simulink library "SignalGeneratorLibBtc"  (R2022b)
settings: Solver=VariableStepAuto  StartTime=0.0  StopTime=10.0  RelTol=1e-3
libraries: simulink x16, FeaturePath x6, HandyTextFile x6, RTC x6, TuneVar x1
(part 2 of 2)

== system SignalGeneratorLibBtc/WhiteNoiseGen/ForEachSubsystem/SimulationTimeTriggered_Subsystem ==
  Constant : Constant  SampleTime=-1
  Digital Clock : DigitalClock  SampleTime=-1
  Equal : RelationalOperator  Operator===  OutDataTypeStr=boolean  RndMeth=Simplest  InputSameDT=off
  SimuliationTimeTriggerdOut1 : Outport  VectorParamsAs1DForOutWhenUnconnected=off
  wires:
  Equal/1 -> SimuliationTimeTriggerdOut1/1
  Constant/1 -> Equal/1
  Digital Clock/1 -> Equal/2

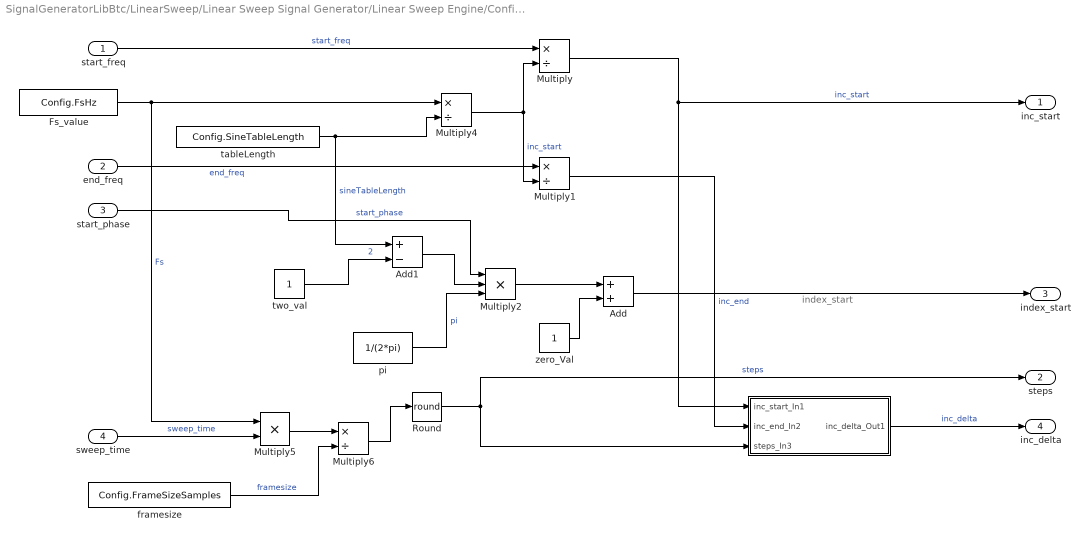
== system SignalGeneratorLibBtc/LinearSweep/Linear Sweep Signal Generator/Linear Sweep Engine/Configuration_sublock ==
  note: index_start
  start_freq : Inport
  end_freq : Inport  Port=2
  start_phase : Inport  Port=3
  "sweep_time " : Inport  Port=4
  " " : Subsystem  TreatAsAtomicUnit=on
  Add : Sum
  Add1 : Sum  Inputs=+-
  Fs_value : Constant  Value=Config.FsHz  OutDataTypeStr=single
  Multiply{,1,4,6} (4 alike) : Product  Inputs=*/
  Multiply2 : Product  Inputs=***
  Multiply5 : Product  Inputs=**
  Round : Rounding  Operator=round
  framesize : Constant  Value=Config.FrameSizeSamples  VectorParams1D=off  OutDataTypeStr=uint32
  pi : Constant  Value=1/(2*pi)  VectorParams1D=off  OutDataTypeStr=single
  tableLength : Constant  Value=Config.SineTableLength  VectorParams1D=off  OutDataTypeStr=single
  two_val : Constant  VectorParams1D=off  OutDataTypeStr=uint32
  zero_Val : Constant  VectorParams1D=off  OutDataTypeStr=single
  inc_start : Outport  VectorParamsAs1DForOutWhenUnconnected=off
  steps : Outport  Port=2  VectorParamsAs1DForOutWhenUnconnected=off
  index_start : Outport  Port=3  VectorParamsAs1DForOutWhenUnconnected=off
  inc_delta : Outport  Port=4  VectorParamsAs1DForOutWhenUnconnected=off
  wires:
  " "/1(inc_delta_Out1) -> inc_delta/1  "inc_delta"
  Round/1 -> steps/1, " "/3(steps_In3)  "steps"
  Multiply6/1 -> Round/1
  framesize/1 -> Multiply6/2  "framesize"
  Multiply5/1 -> Multiply6/1
  "sweep_time "/1 -> Multiply5/2  "sweep_time"
  Multiply1/1 -> " "/2(inc_end_In2)  "inc_end"
  Multiply4/1 -> Multiply/2, Multiply1/2  "inc_start"
  Multiply/1 -> inc_start/1, " "/1(inc_start_In1)  "inc_start"
  Add/1 -> index_start/1
  end_freq/1 -> Multiply1/1  "end_freq"
  start_phase/1 -> Multiply2/1  "start_phase"
  start_freq/1 -> Multiply/1  "start_freq"
  tableLength/1 -> Add1/1, Multiply4/2  "sineTableLength"
  Multiply2/1 -> Add/1
  Fs_value/1 -> Multiply4/1, Multiply5/1  "Fs"
  pi/1 -> Multiply2/3  "pi"
  two_val/1 -> Add1/2  "2"
  zero_Val/1 -> Add/2
  Add1/1 -> Multiply2/2

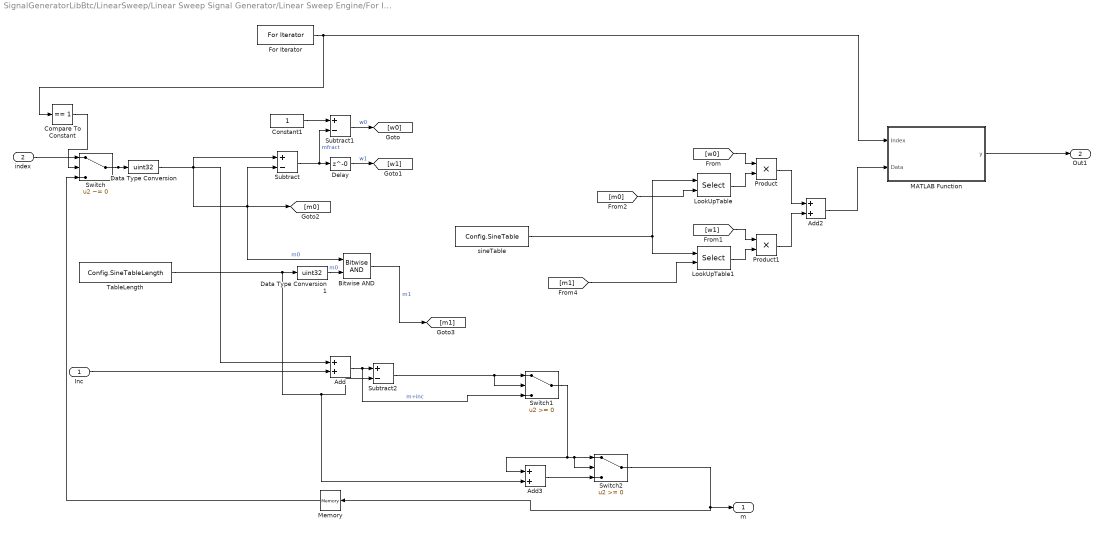
== system SignalGeneratorLibBtc/LinearSweep/Linear Sweep Signal Generator/Linear Sweep Engine/For Iterator Subsystem ==
  "Inc " : Inport
  index : Inport  Port=2
  Add : Sum
  Add2 : Sum
  Add3 : Sum
  Bitwise AND : simulink/Logic and Bit Operations/Bitwise Operator  logicop=AND  UseBitMask=off  NumInputPorts=2  BitMask=bin2dec('11011001')  BitMaskRealWorld=Stored Integer
  Compare To Constant : simulink/Logic and Bit Operations/Compare To Constant  relop===  const=1  OutDataTypeStr=boolean
  Constant1 : Constant  OutDataTypeStr=single
  Data Type Conversion : DataTypeConversion  OutDataTypeStr=uint32  SaturateOnIntegerOverflow=off  RndMeth=Floor
  Data Type Conversion1 : DataTypeConversion  OutDataTypeStr=uint32  SaturateOnIntegerOverflow=off  RndMeth=Floor
  Delay : Delay  DelayLength=0
  For Iterator : ForIterator  ResetStates=reset  IterationLimit=Config.FrameSizeSamples
  LookUpTable : Selector  IndexMode=Zero-based  InputPortWidth=Config.SineTableLength  IndexOptions=Index vector (port)  Indices=[1 3]  OutputSizes=1
  LookUpTable1 : Selector  IndexMode=Zero-based  InputPortWidth=Config.SineTableLength  IndexOptions=Index vector (port)  Indices=[1 3]  OutputSizes=1
  MATLAB Function : MATLAB Function  TreatAsAtomicUnit=on  mask{Nch=Config.NumChannel, frameSize_samples=Config.FrameSizeSamples}
  Memory : Memory  InheritSampleTime=on
  Product : Product
  Product1 : Product
  Subtract : Sum  Inputs=+-  OutDataTypeStr=single
  Subtract1 : Sum  Inputs=+-  OutDataTypeStr=single
  Subtract2 : Sum  Inputs=+-
  Switch : Switch  Criteria=u2 ~= 0  SaturateOnIntegerOverflow=off  InputSameDT=off
  Switch1 : Switch  SaturateOnIntegerOverflow=off  InputSameDT=off
  Switch2 : Switch  SaturateOnIntegerOverflow=off  InputSameDT=off
  TableLength : Constant  Value=Config.SineTableLength  VectorParams1D=off  OutDataTypeStr=single
  sineTable : Constant  Value=Config.SineTable  VectorParams1D=off  OutDataTypeStr=single
  m : Outport  VectorParamsAs1DForOutWhenUnconnected=off
  Out1 : Outport  Port=2  VectorParamsAs1DForOutWhenUnconnected=off
  wires:
  TableLength/1 -> Data Type Conversion1/1, Add3/2, Subtract2/2
  Compare To Constant/1 -> Switch/2
  index/1 -> Switch/1
  Switch/1 -> Add/1, Data Type Conversion/1
  Add/1 -> Switch1/3, Subtract2/1  "m+inc"
  For Iterator/1 -> Compare To Constant/1, MATLAB Function/1(Index)
  Memory/1 -> Switch/3
  Data Type Conversion/1 -> Bitwise AND/1, Subtract/2, [m0], Subtract/1  "m0"
  Subtract/1 -> Delay/1, Subtract1/2  "mfract"
  Constant1/1 -> Subtract1/1
  Subtract1/1 -> [w0]  "w0"
  Delay/1 -> [w1]  "w1"
  sineTable/1 -> LookUpTable1/1, LookUpTable/1
  [m0] -> LookUpTable/2
  [w0] -> Product/1
  LookUpTable/1 -> Product/2
  [m1] -> LookUpTable1/2
  [w1] -> Product1/1
  LookUpTable1/1 -> Product1/2
  Product/1 -> Add2/1
  Product1/1 -> Add2/2
  MATLAB Function/1(y) -> Out1/1
  "Inc "/1 -> Add/2
  Data Type Conversion1/1 -> Bitwise AND/2  "m0"
  Switch1/1 -> Add3/1, Switch2/2, Switch2/1
  Switch2/1 -> Memory/1, m/1
  Subtract2/1 -> Switch1/1, Switch1/2
  Add3/1 -> Switch2/3
  Bitwise AND/1 -> [m1]  "m1"
  Add2/1 -> MATLAB Function/2(Data)

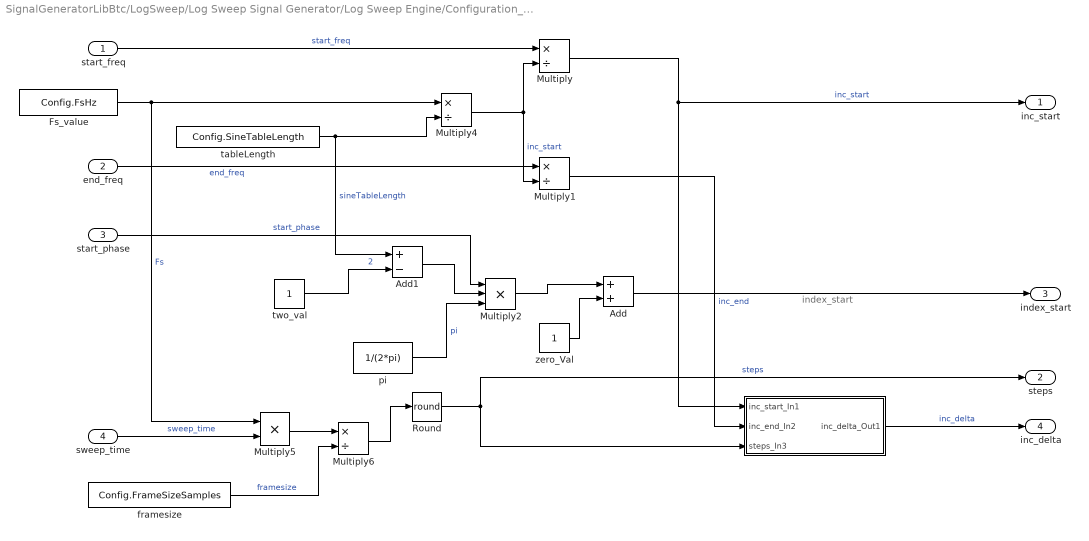
== system SignalGeneratorLibBtc/LogSweep/Log Sweep Signal Generator/Log Sweep Engine/Configuration_sublock ==
  note: index_start
  start_freq : Inport
  end_freq : Inport  Port=2
  start_phase : Inport  Port=3
  "sweep_time " : Inport  Port=4
  " " : Subsystem  AncestorBlock=SignalGenerator/LogSweep/Log Sweep Signal Generator/Log Sweep Engine/Log_Sweep_Subsystem/Configuration_sublock/  TreatAsAtomicUnit=on
      settings: LibrarySourceBlock=SignalGenerator/LogSweep/Log Sweep Signal Generator/Log Sweep Engine/Log_Sweep_Subsystem/Configuration_sublock/
  Add : Sum
  Add1 : Sum  Inputs=+-
  Fs_value : Constant  Value=Config.FsHz  OutDataTypeStr=single
  Multiply{,1,4,6} (4 alike) : Product  Inputs=*/
  Multiply2 : Product  Inputs=***
  Multiply5 : Product  Inputs=**
  Round : Rounding  Operator=round
  framesize : Constant  Value=Config.FrameSizeSamples  VectorParams1D=off  OutDataTypeStr=uint32
  pi : Constant  Value=1/(2*pi)  VectorParams1D=off  OutDataTypeStr=single
  tableLength : Constant  Value=Config.SineTableLength  VectorParams1D=off  OutDataTypeStr=single
  two_val : Constant  VectorParams1D=off  OutDataTypeStr=uint32
  zero_Val : Constant  VectorParams1D=off  OutDataTypeStr=single
  inc_start : Outport  VectorParamsAs1DForOutWhenUnconnected=off
  steps : Outport  Port=2  VectorParamsAs1DForOutWhenUnconnected=off
  index_start : Outport  Port=3  VectorParamsAs1DForOutWhenUnconnected=off
  inc_delta : Outport  Port=4  VectorParamsAs1DForOutWhenUnconnected=off
  wires:
  " "/1(inc_delta_Out1) -> inc_delta/1  "inc_delta"
  Round/1 -> steps/1, " "/3(steps_In3)  "steps"
  Multiply6/1 -> Round/1
  framesize/1 -> Multiply6/2  "framesize"
  Multiply5/1 -> Multiply6/1
  "sweep_time "/1 -> Multiply5/2  "sweep_time"
  Multiply1/1 -> " "/2(inc_end_In2)  "inc_end"
  Multiply4/1 -> Multiply/2, Multiply1/2  "inc_start"
  Multiply/1 -> inc_start/1, " "/1(inc_start_In1)  "inc_start"
  Add/1 -> index_start/1
  end_freq/1 -> Multiply1/1  "end_freq"
  start_freq/1 -> Multiply/1  "start_freq"
  Multiply2/1 -> Add/1
  Fs_value/1 -> Multiply4/1, Multiply5/1  "Fs"
  zero_Val/1 -> Add/2
  Add1/1 -> Multiply2/2
  pi/1 -> Multiply2/3  "pi"
  two_val/1 -> Add1/2  "2"
  tableLength/1 -> Add1/1, Multiply4/2  "sineTableLength"
  start_phase/1 -> Multiply2/1  "start_phase"

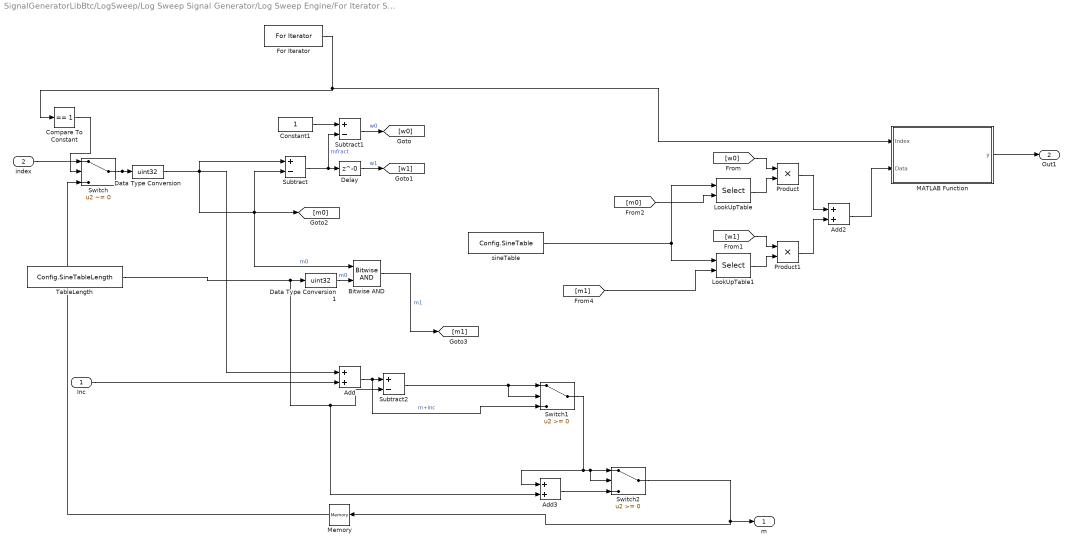
== system SignalGeneratorLibBtc/LogSweep/Log Sweep Signal Generator/Log Sweep Engine/For Iterator Subsystem ==
  "Inc " : Inport
  index : Inport  Port=2
  Add : Sum
  Add2 : Sum
  Add3 : Sum
  Bitwise AND : simulink/Logic and Bit Operations/Bitwise Operator  logicop=AND  UseBitMask=off  NumInputPorts=2  BitMask=bin2dec('11011001')  BitMaskRealWorld=Stored Integer
  Compare To Constant : simulink/Logic and Bit Operations/Compare To Constant  relop===  const=1  OutDataTypeStr=boolean
  Constant1 : Constant  OutDataTypeStr=single
  Data Type Conversion : DataTypeConversion  OutDataTypeStr=uint32  SaturateOnIntegerOverflow=off  RndMeth=Floor
  Data Type Conversion1 : DataTypeConversion  OutDataTypeStr=uint32  SaturateOnIntegerOverflow=off  RndMeth=Floor
  Delay : Delay  DelayLength=0
  For Iterator : ForIterator  ResetStates=reset  IterationLimit=Config.FrameSizeSamples
  LookUpTable : Selector  IndexMode=Zero-based  InputPortWidth=Config.SineTableLength  IndexOptions=Index vector (port)  Indices=[1 3]  OutputSizes=1
  LookUpTable1 : Selector  IndexMode=Zero-based  InputPortWidth=Config.SineTableLength  IndexOptions=Index vector (port)  Indices=[1 3]  OutputSizes=1
  MATLAB Function : MATLAB Function  TreatAsAtomicUnit=on  mask{Nch=Config.NumChannel, frameSize_samples=Config.FrameSizeSamples}
  Memory : Memory  InheritSampleTime=on
  Product : Product
  Product1 : Product
  Subtract : Sum  Inputs=+-  OutDataTypeStr=single
  Subtract1 : Sum  Inputs=+-  OutDataTypeStr=single
  Subtract2 : Sum  Inputs=+-
  Switch : Switch  Criteria=u2 ~= 0  SaturateOnIntegerOverflow=off  InputSameDT=off
  Switch1 : Switch  SaturateOnIntegerOverflow=off  InputSameDT=off
  Switch2 : Switch  SaturateOnIntegerOverflow=off  InputSameDT=off
  TableLength : Constant  Value=Config.SineTableLength  VectorParams1D=off  OutDataTypeStr=single
  sineTable : Constant  Value=Config.SineTable  VectorParams1D=off  OutDataTypeStr=single
  m : Outport  VectorParamsAs1DForOutWhenUnconnected=off
  Out1 : Outport  Port=2  VectorParamsAs1DForOutWhenUnconnected=off
  wires:
  TableLength/1 -> Data Type Conversion1/1, Add3/2, Subtract2/2
  Compare To Constant/1 -> Switch/2
  index/1 -> Switch/1
  Switch/1 -> Add/1, Data Type Conversion/1
  Add/1 -> Switch1/3, Subtract2/1  "m+inc"
  For Iterator/1 -> MATLAB Function/1(Index), Compare To Constant/1
  Memory/1 -> Switch/3
  Data Type Conversion/1 -> Bitwise AND/1, Subtract/2, [m0], Subtract/1  "m0"
  Subtract/1 -> Delay/1, Subtract1/2  "mfract"
  Constant1/1 -> Subtract1/1
  Subtract1/1 -> [w0]  "w0"
  Delay/1 -> [w1]  "w1"
  sineTable/1 -> LookUpTable1/1, LookUpTable/1
  [m0] -> LookUpTable/2
  [w0] -> Product/1
  LookUpTable/1 -> Product/2
  [m1] -> LookUpTable1/2
  [w1] -> Product1/1
  LookUpTable1/1 -> Product1/2
  Product/1 -> Add2/1
  Product1/1 -> Add2/2
  MATLAB Function/1(y) -> Out1/1
  "Inc "/1 -> Add/2
  Data Type Conversion1/1 -> Bitwise AND/2  "m0"
  Switch1/1 -> Add3/1, Switch2/2, Switch2/1
  Switch2/1 -> Memory/1, m/1
  Subtract2/1 -> Switch1/1, Switch1/2
  Add3/1 -> Switch2/3
  Bitwise AND/1 -> [m1]  "m1"
  Add2/1 -> MATLAB Function/2(Data)

== system SignalGeneratorLibBtc/MultiToneGen/Multitone Signal Generator/Multitone Engine/Configuration_sublock ==
  note: index_start
  start_freq : Inport
  start_phase : Inport  Port=2
  Add : Sum
  Fs_value : Constant  Value=Config.FsHz  OutDataTypeStr=single
  Incdelta : Constant  Value=0  OutDataTypeStr=uint32
  Multiply : Product  Inputs=*/
  Multiply1 : Product  Inputs=***
  Multiply4 : Product  Inputs=*/
  Subtract : Sum  Inputs=+-
  constant2 : Constant  OutDataTypeStr=uint32
  tableLength : Constant  Value=Config.SineTableLength  OutDataTypeStr=single
  two_val : Constant  Value=1/(2*pi)  OutDataTypeStr=single
  inc_start : Outport  VectorParamsAs1DForOutWhenUnconnected=off
  index_start : Outport  Port=2  VectorParamsAs1DForOutWhenUnconnected=off
  inc_delta : Outport  Port=3  VectorParamsAs1DForOutWhenUnconnected=off
  wires:
  Incdelta/1 -> inc_delta/1  "inc_delta"
  Multiply4/1 -> Multiply/2
  Multiply/1 -> inc_start/1  "inc_start"
  Add/1 -> index_start/1
  start_phase/1 -> Multiply1/1  "start_phase"
  start_freq/1 -> Multiply/1  "start_freq"
  Multiply1/1 -> Add/1
  tableLength/1 -> Subtract/1, Multiply4/2  "sineTableLength"
  Fs_value/1 -> Multiply4/1  "Fs"
  two_val/1 -> Multiply1/3  "2"
  constant2/1 -> Add/2, Subtract/2
  Subtract/1 -> Multiply1/2

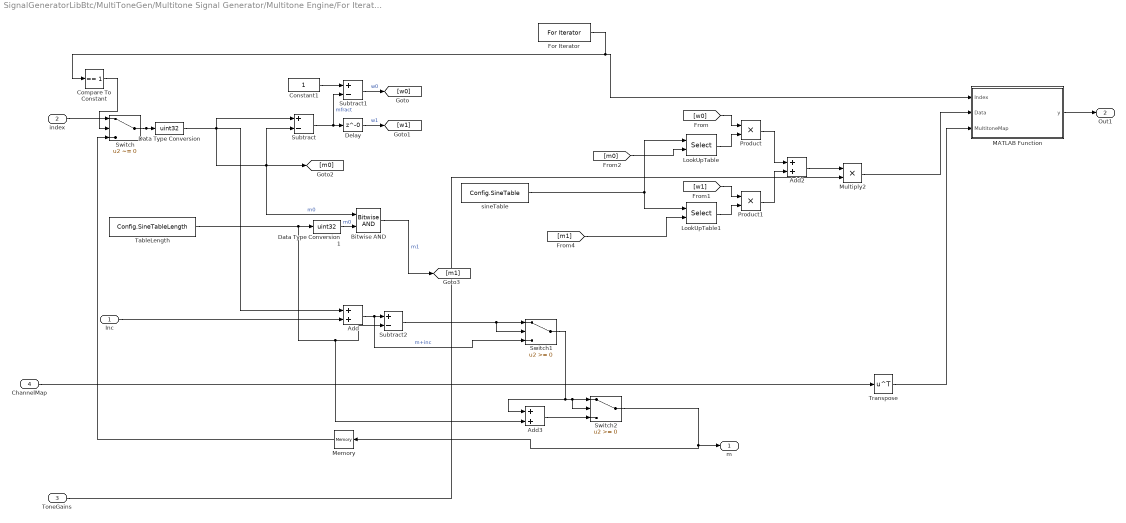
== system SignalGeneratorLibBtc/MultiToneGen/Multitone Signal Generator/Multitone Engine/For Iterator Subsystem ==
  "Inc " : Inport
  index : Inport  Port=2
  ToneGains : Inport  Port=3
  ChannelMap : Inport  Port=4
  Add : Sum
  Add2 : Sum
  Add3 : Sum
  Bitwise AND : simulink/Logic and Bit Operations/Bitwise Operator  logicop=AND  UseBitMask=off  NumInputPorts=2  BitMask=bin2dec('11011001')  BitMaskRealWorld=Stored Integer
  Compare To Constant : simulink/Logic and Bit Operations/Compare To Constant  relop===  const=1  OutDataTypeStr=boolean
  Constant1 : Constant  OutDataTypeStr=single
  Data Type Conversion : DataTypeConversion  OutDataTypeStr=uint32  SaturateOnIntegerOverflow=off  RndMeth=Floor
  Data Type Conversion1 : DataTypeConversion  OutDataTypeStr=uint32  SaturateOnIntegerOverflow=off  RndMeth=Floor
  Delay : Delay  DelayLength=0
  For Iterator : ForIterator  ResetStates=reset  IterationLimit=Config.FrameSizeSamples
  LookUpTable : Selector  IndexMode=Zero-based  InputPortWidth=Config.SineTableLength  IndexOptions=Index vector (port)  Indices=[1 3]  OutputSizes=1
  LookUpTable1 : Selector  IndexMode=Zero-based  InputPortWidth=Config.SineTableLength  IndexOptions=Index vector (port)  Indices=[1 3]  OutputSizes=1
  MATLAB Function : MATLAB Function  TreatAsAtomicUnit=on  mask{frameSize_samples=Config.FrameSizeSamples, Num_Multitone_channels=Config.NumMultitoneChannels}
  Memory : Memory  InheritSampleTime=on
  Multiply2 : Product
  Product : Product
  Product1 : Product
  Subtract : Sum  Inputs=+-  OutDataTypeStr=single
  Subtract1 : Sum  Inputs=+-  OutDataTypeStr=single
  Subtract2 : Sum  Inputs=+-
  Switch : Switch  Criteria=u2 ~= 0  SaturateOnIntegerOverflow=off  InputSameDT=off
  Switch1 : Switch  SaturateOnIntegerOverflow=off  InputSameDT=off
  Switch2 : Switch  SaturateOnIntegerOverflow=off  InputSameDT=off
  TableLength : Constant  Value=Config.SineTableLength  VectorParams1D=off  OutDataTypeStr=single
  Transpose : Math  Operator=transpose  SignedPower=on
  sineTable : Constant  Value=Config.SineTable  VectorParams1D=off  OutDataTypeStr=single
  m : Outport  VectorParamsAs1DForOutWhenUnconnected=off
  Out1 : Outport  Port=2  VectorParamsAs1DForOutWhenUnconnected=off
  wires:
  Transpose/1 -> MATLAB Function/3(MultitoneMap)
  Bitwise AND/1 -> [m1]  "m1"
  Add3/1 -> Switch2/3
  Subtract2/1 -> Switch1/2, Switch1/1
  Switch2/1 -> m/1, Memory/1
  Switch1/1 -> Switch2/1, Switch2/2, Add3/1
  Data Type Conversion1/1 -> Bitwise AND/2  "m0"
  "Inc "/1 -> Add/2
  ToneGains/1 -> Multiply2/2
  Add2/1 -> Multiply2/1
  MATLAB Function/1(y) -> Out1/1
  Product1/1 -> Add2/2
  Product/1 -> Add2/1
  LookUpTable1/1 -> Product1/2
  [w1] -> Product1/1
  [m1] -> LookUpTable1/2
  LookUpTable/1 -> Product/2
  [w0] -> Product/1
  [m0] -> LookUpTable/2
  sineTable/1 -> LookUpTable/1, LookUpTable1/1
  Delay/1 -> [w1]  "w1"
  Subtract1/1 -> [w0]  "w0"
  Constant1/1 -> Subtract1/1
  Subtract/1 -> Subtract1/2, Delay/1  "mfract"
  Data Type Conversion/1 -> Subtract/1, [m0], Subtract/2, Bitwise AND/1  "m0"
  Memory/1 -> Switch/3
  For Iterator/1 -> Compare To Constant/1, MATLAB Function/1(Index)
  Add/1 -> Subtract2/1, Switch1/3  "m+inc"
  Switch/1 -> Data Type Conversion/1, Add/1
  index/1 -> Switch/1
  Compare To Constant/1 -> Switch/2
  TableLength/1 -> Subtract2/2, Add3/2, Data Type Conversion1/1
  ChannelMap/1 -> Transpose/1
  Multiply2/1 -> MATLAB Function/2(Data)

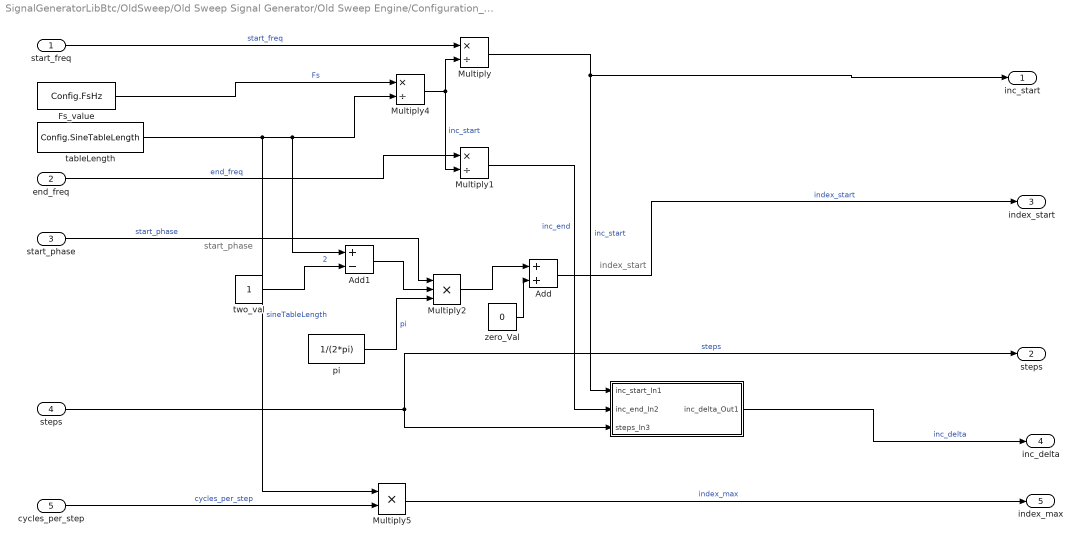
== system SignalGeneratorLibBtc/OldSweep/Old Sweep Signal Generator/Old Sweep Engine/Configuration_sublock ==
  note: start_phase
  note: index_start
  start_freq : Inport
  end_freq : Inport  Port=2
  start_phase : Inport  Port=3
  "steps " : Inport  Port=4
  cycles_per_step : Inport  Port=5
  " " : Subsystem  TreatAsAtomicUnit=on
  Add : Sum
  Add1 : Sum  Inputs=+-
  Fs_value : Constant  Value=Config.FsHz  OutDataTypeStr=single
  Multiply : Product  Inputs=*/
  Multiply1 : Product  Inputs=*/
  Multiply2 : Product  Inputs=***
  Multiply4 : Product  Inputs=*/
  Multiply5 : Product  Inputs=**
  pi : Constant  Value=1/(2*pi)  VectorParams1D=off  OutDataTypeStr=single
  tableLength : Constant  Value=Config.SineTableLength  OutDataTypeStr=single
  two_val : Constant  VectorParams1D=off  OutDataTypeStr=uint32
  zero_Val : Constant  Value=0  OutDataTypeStr=uint32
  inc_start : Outport  VectorParamsAs1DForOutWhenUnconnected=off
  steps : Outport  Port=2  VectorParamsAs1DForOutWhenUnconnected=off
  index_start : Outport  Port=3  VectorParamsAs1DForOutWhenUnconnected=off
  inc_delta : Outport  Port=4  VectorParamsAs1DForOutWhenUnconnected=off
  index_max : Outport  Port=5  VectorParamsAs1DForOutWhenUnconnected=off
  wires:
  zero_Val/1 -> Add/2
  Fs_value/1 -> Multiply4/1  "Fs"
  Multiply2/1 -> Add/1
  start_freq/1 -> Multiply/1  "start_freq"
  end_freq/1 -> Multiply1/1  "end_freq"
  Multiply/1 -> " "/1(inc_start_In1), inc_start/1  "inc_start"
  Multiply4/1 -> Multiply1/2, Multiply/2  "inc_start"
  Multiply1/1 -> " "/2(inc_end_In2)  "inc_end"
  "steps "/1 -> steps/1, " "/3(steps_In3)  "steps"
  " "/1(inc_delta_Out1) -> inc_delta/1  "inc_delta"
  Multiply5/1 -> index_max/1  "index_max"
  cycles_per_step/1 -> Multiply5/2  "cycles_per_step"
  Add/1 -> index_start/1  "index_start"
  Add1/1 -> Multiply2/2
  pi/1 -> Multiply2/3  "pi"
  two_val/1 -> Add1/2  "2"
  tableLength/1 -> Add1/1, Multiply4/2, Multiply5/1  "sineTableLength"
  start_phase/1 -> Multiply2/1  "start_phase"

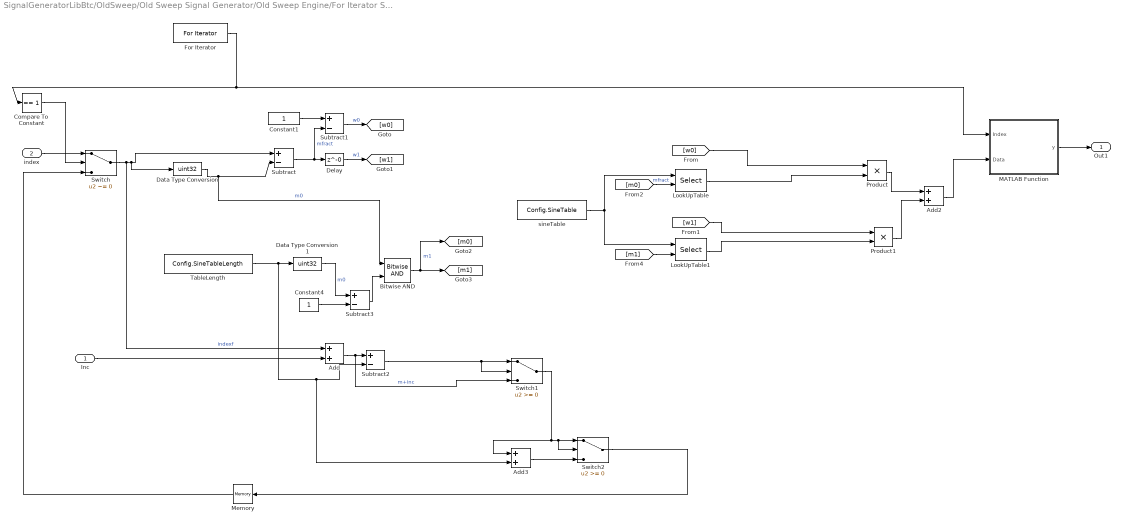
== system SignalGeneratorLibBtc/OldSweep/Old Sweep Signal Generator/Old Sweep Engine/For Iterator Subsystem ==
  "Inc " : Inport
  index : Inport  Port=2
  Add : Sum
  Add2 : Sum
  Add3 : Sum
  Bitwise AND : simulink/Logic and Bit Operations/Bitwise Operator  logicop=AND  UseBitMask=off  NumInputPorts=2  BitMask=bin2dec('11011001')  BitMaskRealWorld=Stored Integer
  Compare To Constant : simulink/Logic and Bit Operations/Compare To Constant  relop===  const=1  OutDataTypeStr=boolean
  Constant1 : Constant  OutDataTypeStr=single
  Constant4 : Constant  OutDataTypeStr=uint32
  Data Type Conversion : DataTypeConversion  OutDataTypeStr=uint32  SaturateOnIntegerOverflow=off  RndMeth=Floor
  Data Type Conversion1 : DataTypeConversion  OutDataTypeStr=uint32  SaturateOnIntegerOverflow=off  RndMeth=Floor
  Delay : Delay  DelayLength=0
  For Iterator : ForIterator  ResetStates=reset  IterationLimit=Config.FrameSizeSamples
  LookUpTable : Selector  IndexMode=Zero-based  InputPortWidth=Config.SineTableLength  IndexOptions=Index vector (port)  Indices=[1 3]  OutputSizes=1
  LookUpTable1 : Selector  IndexMode=Zero-based  InputPortWidth=Config.SineTableLength  IndexOptions=Index vector (port)  Indices=[1 3]  OutputSizes=1
  MATLAB Function : MATLAB Function  TreatAsAtomicUnit=on  mask{Nch=Config.NumChannel, frameSize_samples=Config.FrameSizeSamples}
  Memory : Memory  InheritSampleTime=on
  Product : Product
  Product1 : Product
  Subtract : Sum  Inputs=+-  OutDataTypeStr=single
  Subtract1 : Sum  Inputs=+-  OutDataTypeStr=single
  Subtract2 : Sum  Inputs=+-
  Subtract3 : Sum  Inputs=+-
  Switch : Switch  Criteria=u2 ~= 0  SaturateOnIntegerOverflow=off  InputSameDT=off
  Switch1 : Switch  SaturateOnIntegerOverflow=off  InputSameDT=off
  Switch2 : Switch  SaturateOnIntegerOverflow=off  InputSameDT=off
  TableLength : Constant  Value=Config.SineTableLength  VectorParams1D=off  OutDataTypeStr=single
  sineTable : Constant  Value=Config.SineTable  VectorParams1D=off  OutDataTypeStr=single
  Out1 : Outport  VectorParamsAs1DForOutWhenUnconnected=off
  wires:
  [m0] -> LookUpTable/2  "mfract"
  Constant4/1 -> Subtract3/2
  Subtract3/1 -> Bitwise AND/2
  Data Type Conversion1/1 -> Subtract3/1  "m0"
  Add2/1 -> MATLAB Function/2(Data)
  TableLength/1 -> Data Type Conversion1/1, Add3/2, Subtract2/2
  Compare To Constant/1 -> Switch/2
  index/1 -> Switch/1
  Switch/1 -> Add/1, Subtract/1, Data Type Conversion/1  "indexf"
  Add/1 -> Switch1/3, Subtract2/1  "m+inc"
  For Iterator/1 -> Compare To Constant/1, MATLAB Function/1(Index)
  Memory/1 -> Switch/3
  Data Type Conversion/1 -> Bitwise AND/1, Subtract/2  "m0"
  Subtract/1 -> Delay/1, Subtract1/2  "mfract"
  Constant1/1 -> Subtract1/1
  Subtract1/1 -> [w0]  "w0"
  Delay/1 -> [w1]  "w1"
  sineTable/1 -> LookUpTable/1, LookUpTable1/1
  [w0] -> Product/1
  LookUpTable/1 -> Product/2
  [m1] -> LookUpTable1/2
  [w1] -> Product1/1
  LookUpTable1/1 -> Product1/2
  Product/1 -> Add2/1
  Product1/1 -> Add2/2
  MATLAB Function/1(y) -> Out1/1
  "Inc "/1 -> Add/2
  Switch1/1 -> Add3/1, Switch2/2, Switch2/1
  Switch2/1 -> Memory/1
  Subtract2/1 -> Switch1/1, Switch1/2
  Add3/1 -> Switch2/3
  Bitwise AND/1 -> [m1], [m0]  "m1"

== system SignalGeneratorLibBtc/Sawtooth/SawtoothGenSubsystem/Subsystem/Disable_Sawtooth ==
  Action Port : ActionPort
  SawtoothZeroOut : MATLAB Function  TreatAsAtomicUnit=on  mask{Nch=Config.NumChannel, frameSize_samples=Config.FrameSizeSamples}
  Output : Outport  VectorParamsAs1DForOutWhenUnconnected=off
  wires:
  SawtoothZeroOut/1(y) -> Output/1

== system SignalGeneratorLibBtc/Sawtooth/SawtoothGenSubsystem/Subsystem/SigGen_Sawtooth ==
  StartFreq : Inport
  start_phase : Inport  Port=2
  Action Port : ActionPort
  Add3 : Sum
  Divide2 : Product  Inputs=*/
  For Iterator Subsystem : Subsystem  TreatAsAtomicUnit=on
  Mod2 : Math  Operator=mod  SignedPower=on
  module_phase1 : Constant  Value=1.0  OutDataTypeStr=single
  sampling_frequency : Constant  Value=Config.FsHz  OutDataTypeStr=single  SampleTime=Inf
  sawtooth_offset1 : Constant  Value=0.5  OutDataTypeStr=single
  Output1 : Outport  VectorParamsAs1DForOutWhenUnconnected=off
  wires:
  StartFreq/1 -> Divide2/1
  For Iterator Subsystem/1(Out1) -> Output1/1
  sampling_frequency/1 -> Divide2/2
  Mod2/1 -> Add3/1  "initial_phase"
  module_phase1/1 -> For Iterator Subsystem/4(ModulePhase), Mod2/2
  start_phase/1 -> Mod2/1
  Divide2/1 -> For Iterator Subsystem/3(IncStart)  "inc_start"
  Add3/1 -> For Iterator Subsystem/1(IndexStart)  "index_start"
  sawtooth_offset1/1 -> Add3/2, For Iterator Subsystem/2(SawtoothOffset)

== system SignalGeneratorLibBtc/WhiteNoiseGen/ForEachSubsystem/SigGen_Noise/For Iterator Subsystem ==
  InitSeed : Inport
  Add1 : Sum
  Constant2 : Constant  Value=4.656612873077393e-010
  Constant3 : Constant  Value=1664525
  Constant4 : Constant
  Constant5 : Constant  Value=1013904223
  Data Type Conversion : DataTypeConversion  OutDataTypeStr=uint32  SaturateOnIntegerOverflow=off  RndMeth=Floor
  Delay1 : Delay  DelayLength=1  InitialConditionSource=Input port
      settings: InputPortMap=u0,p4
  For Iterator : ForIterator  IterationLimit=Config.FrameSizeSamples
  MATLAB Function : MATLAB Function  TreatAsAtomicUnit=on  mask{Nch=Config.NumChannel, frameSize_samples=Config.FrameSizeSamples}
  Multiply : Product
  Multiply1 : Product
  Subtract : Sum  Inputs=+-
  noiseOut1 : Outport  VectorParamsAs1DForOutWhenUnconnected=off
  wires:
  InitSeed/1 -> Delay1/2
  Delay1/1 -> Data Type Conversion/1
  Add1/1 -> Delay1/1
  Constant5/1 -> Add1/2
  Multiply1/1 -> Add1/1
  Subtract/1 -> MATLAB Function/2(Data)
  Constant4/1 -> Subtract/2
  Constant3/1 -> Multiply1/2
  Multiply/1 -> Subtract/1
  Constant2/1 -> Multiply/1
  Data Type Conversion/1 -> Multiply/2, Multiply1/1
  For Iterator/1 -> MATLAB Function/1(Index)
  MATLAB Function/1(y) -> noiseOut1/1

== system SignalGeneratorLibBtc/LinearSweep/Linear Sweep Signal Generator/Linear Sweep Engine/Configuration_sublock/  ==
  inc_start_In1 : Inport
  inc_end_In2 : Inport  Port=2
  steps_In3 : Inport  Port=3
  Add : Sum  Inputs=+-
  Multiply1 : Product  Inputs=*/
  inc_delta_Out1 : Outport  VectorParamsAs1DForOutWhenUnconnected=off
  wires:
  steps_In3/1 -> Multiply1/2  "steps"
  Multiply1/1 -> inc_delta_Out1/1
  Add/1 -> Multiply1/1
  inc_end_In2/1 -> Add/1  "inc_end"
  inc_start_In1/1 -> Add/2  "inc_start"

== system SignalGeneratorLibBtc/LogSweep/Log Sweep Signal Generator/Log Sweep Engine/Configuration_sublock/  ==
  inc_start_In1 : Inport
  inc_end_In2 : Inport  Port=2
  steps_In3 : Inport  Port=3
  Math Function : Math  Operator=pow  SignedPower=on
  Multiply : Product  Inputs=*/
  Multiply1 : Product  Inputs=*/
  oneVal : Constant  OutDataTypeStr=single
  inc_delta_Out1 : Outport  VectorParamsAs1DForOutWhenUnconnected=off
  wires:
  inc_start_In1/1 -> Multiply/2  "inc_start"
  inc_end_In2/1 -> Multiply/1  "inc_end"
  Math Function/1 -> inc_delta_Out1/1  "inc_delta"
  steps_In3/1 -> Multiply1/2  "steps"
  oneVal/1 -> Multiply1/1  "1"
  Multiply/1 -> Math Function/1
  Multiply1/1 -> Math Function/2

== system SignalGeneratorLibBtc/OldSweep/Old Sweep Signal Generator/Old Sweep Engine/Configuration_sublock/  ==
  inc_start_In1 : Inport
  inc_end_In2 : Inport  Port=2
  steps_In3 : Inport  Port=3
  Add : Sum  Inputs=+-
  Multiply1 : Product  Inputs=*/
  Subtract : Sum  Inputs=+-
  oneVal : Constant  OutDataTypeStr=uint32
  inc_delta_Out1 : Outport  VectorParamsAs1DForOutWhenUnconnected=off
  wires:
  inc_start_In1/1 -> Add/2  "inc_start"
  inc_end_In2/1 -> Add/1  "inc_end"
  Add/1 -> Multiply1/1
  Multiply1/1 -> inc_delta_Out1/1
  steps_In3/1 -> Subtract/1  "steps_state"
  oneVal/1 -> Subtract/2
  Subtract/1 -> Multiply1/2

== system SignalGeneratorLibBtc/Sawtooth/SawtoothGenSubsystem/Subsystem/SigGen_Sawtooth/For Iterator Subsystem ==
  IndexStart : Inport
  SawtoothOffset : Inport  Port=2
  IncStart : Inport  Port=3
  ModulePhase : Inport  Port=4
  Add1 : Sum
  Constant : Constant  Value=-2.0  OutDataTypeStr=single
  Delay : Delay  DelayLength=1  InitialConditionSource=Input port
      settings: InputPortMap=u0,p4
  For Iterator : ForIterator  IterationLimit=Config.FrameSizeSamples
  MATLAB Function : MATLAB Function  TreatAsAtomicUnit=on  mask{Nch=Config.NumChannel, frameSize_samples=Config.FrameSizeSamples}
  Mod1 : Math  Operator=mod  SignedPower=on
  Multiply : Product
  Subtract : Sum  Inputs=+-
  Out1 : Outport  VectorParamsAs1DForOutWhenUnconnected=off
  wires:
  For Iterator/1 -> MATLAB Function/1(Index)
  Multiply/1 -> MATLAB Function/2(Data)
  Mod1/1 -> Delay/1  "initial_phase"
  Add1/1 -> Mod1/1
  Constant/1 -> Multiply/2
  Subtract/1 -> Multiply/1
  Delay/1 -> Add1/1, Subtract/1  "phase"
  IncStart/1 -> Add1/2  "inc_start"
  IndexStart/1 -> Delay/2  "index_start"
  SawtoothOffset/1 -> Subtract/2
  ModulePhase/1 -> Mod1/2
  MATLAB Function/1(y) -> Out1/1

== matlab function SignalGeneratorLibBtc/Sawtooth/SawtoothGenSubsystem/Subsystem/Disable_Sawtooth/SawtoothZeroOut ==
  data: y output size=[frameSize_samples, Nch]; frameSize_samples parameter; Nch parameter
function y = fcn(frameSize_samples, Nch)
% zero out when sawtooth not in use
y = single(zeros(frameSize_samples,Nch));

== matlab function SignalGeneratorLibBtc/WhiteNoiseGen/ForEachSubsystem/Disable_Noise/RandomNoiseZeroOut ==
  data: y output size=[frameSize_samples, Nch]; frameSize_samples parameter; Nch parameter
function y = fcn(frameSize_samples, Nch)
% zero out when random noise not in use
y = single(zeros(frameSize_samples,Nch));

== matlab function SignalGeneratorLibBtc/MultiToneGen/Multitone Signal Generator/Multitone Engine/MultitoneZeroOut ==
  data: y output size=[frameSize_samples, Num_Multitone_channels]; frameSize_samples parameter; Num_Multitone_channels parameter
function y = fcn(frameSize_samples, Num_Multitone_channels)
% zero out when multitone not in use
y = single(zeros(frameSize_samples,Num_Multitone_channels));

== matlab function SignalGeneratorLibBtc/LogSweep/Log Sweep Signal Generator/Log Sweep Engine/For Iterator Subsystem/MATLAB Function ==
  data: Index input; Data input; y output size=[frameSize_samples, Nch]; frameSize_samples parameter; Nch parameter
function y = fcn(Index,Data, frameSize_samples, Nch)  

% init
persistent OutStore ;
% comment
if(isempty(OutStore))
    OutStore = single(zeros(frameSize_samples,Nch));
end
% fill output
OutStore(Index,1:Nch) = Data';
y = OutStore;

== matlab function SignalGeneratorLibBtc/OldSweep/Old Sweep Signal Generator/Old Sweep Engine/For Iterator Subsystem/MATLAB Function ==
  data: Index input; Data input; y output size=[frameSize_samples, Nch]; frameSize_samples parameter; Nch parameter
function y = fcn(Index, Data,frameSize_samples, Nch)
% init
persistent OutStore ;
% check if empty
if(isempty(OutStore))
   
    OutStore = single(zeros(frameSize_samples,Nch));
end
% fill out data
OutStore(Index,1:Nch) = Data;
y = OutStore;

== matlab function SignalGeneratorLibBtc/WhiteNoiseGen/ForEachSubsystem/SigGen_Noise/For Iterator Subsystem/MATLAB Function ==
  data: Index input; Data input; y output size=[frameSize_samples, Nch]; frameSize_samples parameter; Nch parameter
function y = fcn(Index, Data,frameSize_samples, Nch)
% init
persistent OutStore ;
% check if empty
if(isempty(OutStore))
    % comment
    OutStore = single(zeros(frameSize_samples,Nch));
end
% fill out data
OutStore(Index,1:Nch) = Data;
y = OutStore;

== matlab function SignalGeneratorLibBtc/LinearSweep/Linear Sweep Signal Generator/Linear Sweep Engine/LinearSweepZeroOut ==
  data: y output; frameSize_samples parameter; Nch parameter
function y = fcn(frameSize_samples, Nch)
% output zeros when not in use
y = single(zeros(frameSize_samples,Nch));

== matlab function SignalGeneratorLibBtc/Sawtooth/SawtoothGenSubsystem/Subsystem/SigGen_Sawtooth/For Iterator Subsystem/MATLAB Function ==
  data: Index input; Data input; y output size=[frameSize_samples, Nch]; frameSize_samples parameter; Nch parameter
function y = fcn(Index, Data,frameSize_samples, Nch)
% init
persistent OutStore ;
% comment
if(isempty(OutStore))
    % zeros padding
    OutStore = single(zeros(frameSize_samples,Nch));
end
% comment
OutStore(Index,1:Nch) = Data;
% comment
y = OutStore;

== matlab function SignalGeneratorLibBtc/LinearSweep/Linear Sweep Signal Generator/Linear Sweep Engine/For Iterator Subsystem/MATLAB Function ==
  data: Index input; Data input; y output size=[frameSize_samples Nch]; frameSize_samples parameter; Nch parameter
function y = fcn(Index,Data,frameSize_samples, Nch)

% init
persistent OutStore ;
if(isempty(OutStore))
    % comment
    OutStore = single(zeros(frameSize_samples,Nch));
end
% fill output
OutStore(Index,1:Nch) = Data';
y = OutStore;

== matlab function SignalGeneratorLibBtc/MultiToneGen/Multitone Signal Generator/Multitone Engine/For Iterator Subsystem/MATLAB Function ==
  data: Index input; Data input; y output size=[frameSize_samples, Num_Multitone_channels]; MultitoneMap input; frameSize_samples parameter
function y = fcn(Index,Data,MultitoneMap, frameSize_samples)

% out size
OutChNumSize = size(MultitoneMap,2);
%y = coder.nullcopy(single(zeros(frameSize_samples, Num_Multitone_channels)));
persistent OutStore ;
% init
if(isempty(OutStore))
    OutStore = single(zeros(frameSize_samples,OutChNumSize));
end
for OutChNum = 1:OutChNumSize
    % comment
    ToneSize = MultitoneMap(OutChNum);
    if(OutChNum == 1)
        idx_start = 1;
    else
        idx_start = sum(MultitoneMap(1:OutChNum));
    end
    OutStore(Index,OutChNum) = sum(Data(idx_start:idx_start+ToneSize-1));
end
%OutStore(Index,1:Numchannels) = Data;
y = OutStore;

== matlab function SignalGeneratorLibBtc/LogSweep/Log Sweep Signal Generator/Log Sweep Engine/LogSweepZeroOut ==
  data: y output; frameSize_samples parameter; Nch parameter
function y = fcn(frameSize_samples, Nch)
% zero out when log sweep not in use
y = single(zeros(frameSize_samples,Nch));

== matlab function SignalGeneratorLibBtc/OldSweep/Old Sweep Signal Generator/Old Sweep Engine/OldSweepZeroOut ==
  data: y output; frameSize_samples parameter; Nch parameter
function y = fcn(frameSize_samples, Nch)
% zero out when log sweep not in use
y = single(zeros(frameSize_samples,Nch));
